simulink model "reacwheelfailure"  (R2014a)
settings: Solver=ode45  StartTime=0.0  StopTime=100.0  RelTol=1e-3
undefined symbols (not defined in the file): DiscIntNeverNeededParam, k, q1, q2, q3, q4
libraries: aerolibutil x2
settings Model: Creator=Gokull  LastModifiedBy=Gokull

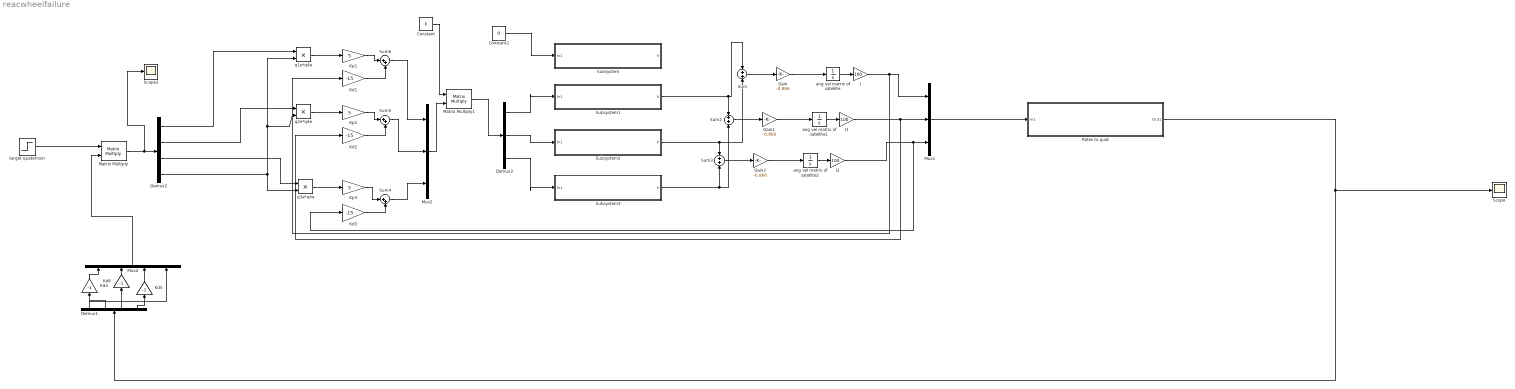
== system reacwheelfailure ==
  Constant : Constant  Value=k
  Constant1 : Constant  Value=0
  Demux1 : Demux
  Demux2 : Demux
  Demux3 : Demux  Outputs=3
  Gain : Gain  Gain=-0.866
  Gain1 : Gain  Gain=-0.866
  Gain2 : Gain  Gain=-0.866
  I : Gain  Gain=100
  I1 : Gain  Gain=100
  I2 : Gain  Gain=100
  Kd1 : Gain  Gain=-15
  Kd2 : Gain  Gain=-15
  Kd3 : Gain  Gain=-15
  Kd4 : Gain  Gain=-1
  Kd5 : Gain  Gain=-1
  Kd6 : Gain  Gain=-1
  Kp1 : Gain  Gain=5
  Kp2 : Gain  Gain=5
  Kp3 : Gain  Gain=5
  Matrix Multiply : Product  Multiplication=Matrix(*)
  Matrix Multiply1 : Product  Multiplication=Matrix(*)
  Mux1 : Mux  Inputs=3
  Mux2 : Mux  Inputs=3
  Mux4 : Mux
  Rates to quat : Subsystem
  Scope : Scope
      settings: TimeRange=600  YMin=-1  YMax=1  SaveName=ScopeData2
  Scope3 : Scope
      settings: SaveName=ScopeData3
  Subsystem : Subsystem
  Subsystem1 : Subsystem
  Subsystem2 : Subsystem
  Subsystem3 : Subsystem
  Sum : Sum  Inputs=+|+
  Sum2 : Sum  Inputs=+|+
  Sum3 : Sum  Inputs=+|+
  Sum4 : Sum  Inputs=|++
  Sum5 : Sum  Inputs=|++
  Sum6 : Sum  Inputs=|++
  ang vel matrix of satellite : Integrator
  ang vel matrix of satellite1 : Integrator
  ang vel matrix of satellite2 : Integrator
  q1e*q4e : Product
  q2e*q4e : Product
  q3e*q4e : Product
  target quaternion : Step  Before=[1,0,0,0;0,1,0,0;0,0,1,0;0,0,0,1]  After=[q4,q3,-q2,q1;-q3,q4,q1,q2;q2,-q1,q4,q3;-q1,-q2,-q3,q4]  SampleTime=0
  wires:
  Demux2/4 -> q1e*q4e/2, q2e*q4e/2, q3e*q4e/2
  q1e*q4e/1 -> Kp1/1
  q2e*q4e/1 -> Kp2/1
  q3e*q4e/1 -> Kp3/1
  Kp1/1 -> Sum6/1
  Kd1/1 -> Sum6/2
  Kp2/1 -> Sum5/1
  Kd2/1 -> Sum5/2
  Kp3/1 -> Sum4/1
  Kd3/1 -> Sum4/2
  Matrix Multiply/1 -> Scope3/1, Demux2/1
  Demux1/2 -> Kd4/1
  Demux1/3 -> Kd6/1
  Demux1/4 -> Kd5/1
  Demux1/1 -> Mux4/4
  target quaternion/1 -> Matrix Multiply/1
  Kd4/1 -> Mux4/1
  Kd6/1 -> Mux4/2
  Kd5/1 -> Mux4/3
  Mux4/1 -> Matrix Multiply/2
  Demux2/1 -> q1e*q4e/1
  Demux2/2 -> q2e*q4e/1
  Demux2/3 -> q3e*q4e/1
  Rates to quat/1(Out1) -> Demux1/1, Scope/1
  Subsystem3/1(h) -> Sum2/2, Sum3/2
  Subsystem1/1(h) -> Sum/1, Sum2/1
  Sum/1 -> Gain/1
  Gain/1 -> ang vel matrix of satellite/1
  ang vel matrix of satellite/1 -> I/1
  Mux1/1 -> Rates to quat/1(In1)
  Sum2/1 -> Gain1/1
  Gain1/1 -> ang vel matrix of satellite1/1
  ang vel matrix of satellite1/1 -> I1/1
  Sum3/1 -> Gain2/1
  Gain2/1 -> ang vel matrix of satellite2/1
  ang vel matrix of satellite2/1 -> I2/1
  Subsystem2/1(h) -> Sum/2, Sum3/1
  I1/1 -> Kd2/1, Mux1/2
  I/1 -> Kd1/1, Mux1/1
  I2/1 -> Kd3/1, Mux1/3
  Sum6/1 -> Mux2/1
  Sum5/1 -> Mux2/2
  Sum4/1 -> Mux2/3
  Constant/1 -> Matrix Multiply1/1
  Mux2/1 -> Matrix Multiply1/2
  Matrix Multiply1/1 -> Demux3/1
  Demux3/1 -> Subsystem1/1(In1)
  Demux3/2 -> Subsystem2/1(In1)
  Demux3/3 -> Subsystem3/1(In1)
  Constant1/1 -> Subsystem/1(In1)

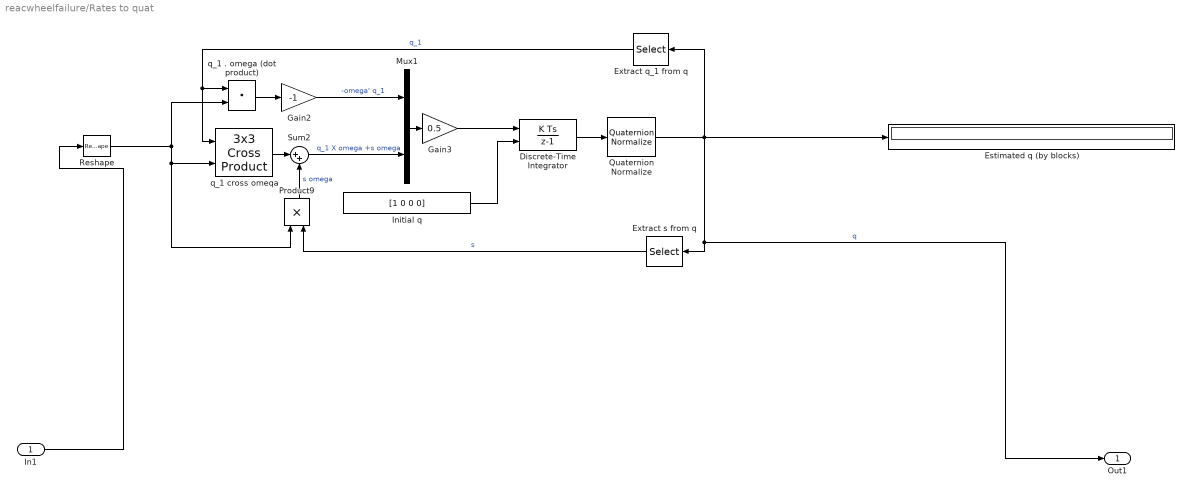
== system reacwheelfailure/Rates to quat ==
  In1 : Inport
  Discrete-Time Integrator : DiscreteIntegrator  InitialConditionSource=external  SampleTime=0.1  ICPrevOutput=DiscIntNeverNeededParam  ICPrevScaledInput=DiscIntNeverNeededParam
  Estimated q (by blocks) : Display
  Extract q_1 from q : Selector  InputPortWidth=4  Indices=[2:4]
  Extract s from q : Selector  InputPortWidth=4
  Gain2 : Gain  Gain=-1  SaturateOnIntegerOverflow=on  OutDataTypeStr=Inherit: Same as input  ParamDataTypeStr=Inherit: Same as input
  Gain3 : Gain  Gain=0.5  SaturateOnIntegerOverflow=on  OutDataTypeStr=Inherit: Same as input  ParamDataTypeStr=Inherit: Same as input
  "Initial q " : Constant  Value=[1 0 0 0]  VectorParams1D=off
  Mux1 : Mux  Inputs=2
  Product9 : Product  Inputs=**  SaturateOnIntegerOverflow=on  InputSameDT=on  OutDataTypeStr=Inherit: Same as first input
  Quaternion Normalize : aerolibutil/Quaternion Normalize
  Reshape : Reshape  OutputDimensionality=Row vector (2-D)
  Sum2 : Sum  Inputs=|++  SaturateOnIntegerOverflow=on
  q_1 . omega (dot product) : DotProduct  InputSameDT=on  OutDataTypeStr=Inherit: Inherit via internal rule
  q_1 cross omeqa : aerolibutil/3x3 Cross Product
  Out1 : Outport
  wires:
  Mux1/1 -> Gain3/1
  Quaternion Normalize/1 -> Out1/1, Extract s from q/1, Estimated q (by blocks)/1, Extract q_1 from q/1  "q"
  "Initial q "/1 -> Discrete-Time Integrator/2
  q_1 . omega (dot product)/1 -> Gain2/1
  Product9/1 -> Sum2/2  "s omega"
  Reshape/1 -> q_1 . omega (dot product)/2, q_1 cross omeqa/2, Product9/1
  q_1 cross omeqa/1 -> Sum2/1
  Sum2/1 -> Mux1/2  "q_1 X omega +s omega"
  Discrete-Time Integrator/1 -> Quaternion Normalize/1
  Gain2/1 -> Mux1/1  "-omega' q_1"
  Extract s from q/1 -> Product9/2  "s"
  Extract q_1 from q/1 -> q_1 cross omeqa/1, q_1 . omega (dot product)/1  "q_1"
  Gain3/1 -> Discrete-Time Integrator/1
  In1/1 -> Reshape/1

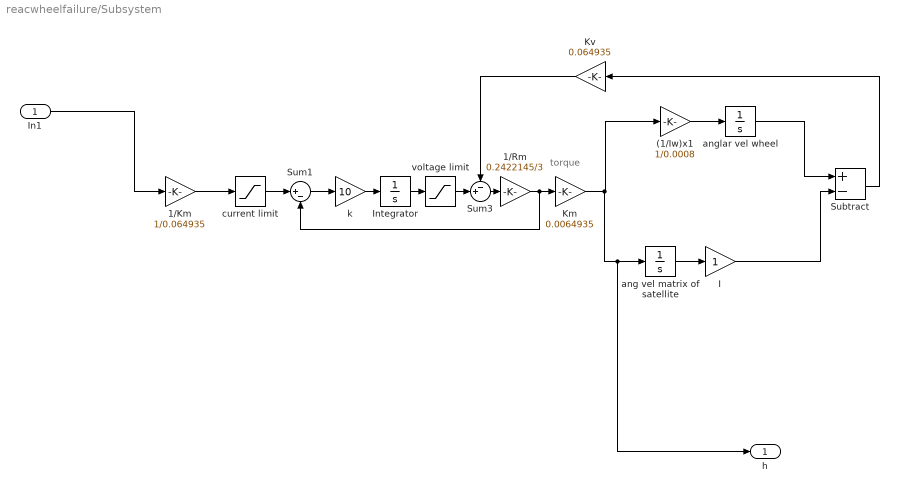
== system reacwheelfailure/Subsystem ==
  note: torque
  In1 : Inport
  (1/Iw)x1 : Gain  Gain=1/0.0008
  1/Km : Gain  Gain=1/0.064935
  1/Rm : Gain  Gain=0.2422145/3
  I : Gain
  Integrator : Integrator
  Km : Gain  Gain=0.0064935
  Kv : Gain  Gain=0.064935
  Subtract : Sum  Inputs=+-
  Sum1 : Sum  Inputs=|+-
  Sum3 : Sum  Inputs=-+|
  ang vel matrix of satellite : Integrator
  anglar vel wheel : Integrator
  current limit : Saturate  UpperLimit=0.8  LowerLimit=-0.8
  k : Gain  Gain=10
  voltage limit : Saturate  UpperLimit=35  LowerLimit=-35
  h : Outport
  wires:
  1/Km/1 -> current limit/1
  k/1 -> Integrator/1
  1/Rm/1 -> Sum1/2, Km/1
  current limit/1 -> Sum1/1
  Sum1/1 -> k/1
  Sum3/1 -> 1/Rm/1
  voltage limit/1 -> Sum3/2
  Integrator/1 -> voltage limit/1
  anglar vel wheel/1 -> Subtract/1
  Subtract/1 -> Kv/1
  I/1 -> Subtract/2
  (1/Iw)x1/1 -> anglar vel wheel/1
  In1/1 -> 1/Km/1
  Km/1 -> h/1, ang vel matrix of satellite/1, (1/Iw)x1/1
  Kv/1 -> Sum3/1
  ang vel matrix of satellite/1 -> I/1

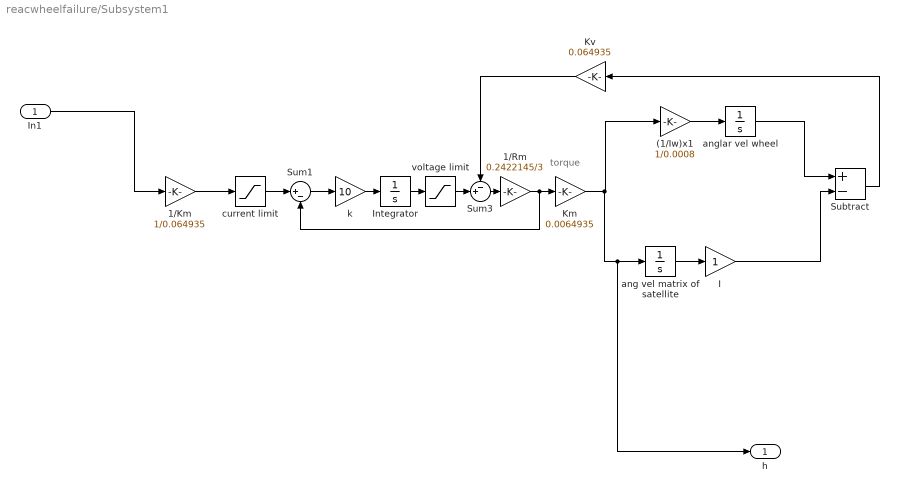
== system reacwheelfailure/Subsystem1 ==
  note: torque
  In1 : Inport
  (1/Iw)x1 : Gain  Gain=1/0.0008
  1/Km : Gain  Gain=1/0.064935
  1/Rm : Gain  Gain=0.2422145/3
  I : Gain
  Integrator : Integrator
  Km : Gain  Gain=0.0064935
  Kv : Gain  Gain=0.064935
  Subtract : Sum  Inputs=+-
  Sum1 : Sum  Inputs=|+-
  Sum3 : Sum  Inputs=-+|
  ang vel matrix of satellite : Integrator
  anglar vel wheel : Integrator
  current limit : Saturate  UpperLimit=0.8  LowerLimit=-0.8
  k : Gain  Gain=10
  voltage limit : Saturate  UpperLimit=35  LowerLimit=-35
  h : Outport
  wires:
  1/Km/1 -> current limit/1
  k/1 -> Integrator/1
  1/Rm/1 -> Sum1/2, Km/1
  current limit/1 -> Sum1/1
  Sum1/1 -> k/1
  Sum3/1 -> 1/Rm/1
  voltage limit/1 -> Sum3/2
  Integrator/1 -> voltage limit/1
  anglar vel wheel/1 -> Subtract/1
  Subtract/1 -> Kv/1
  I/1 -> Subtract/2
  (1/Iw)x1/1 -> anglar vel wheel/1
  In1/1 -> 1/Km/1
  Km/1 -> h/1, ang vel matrix of satellite/1, (1/Iw)x1/1
  Kv/1 -> Sum3/1
  ang vel matrix of satellite/1 -> I/1

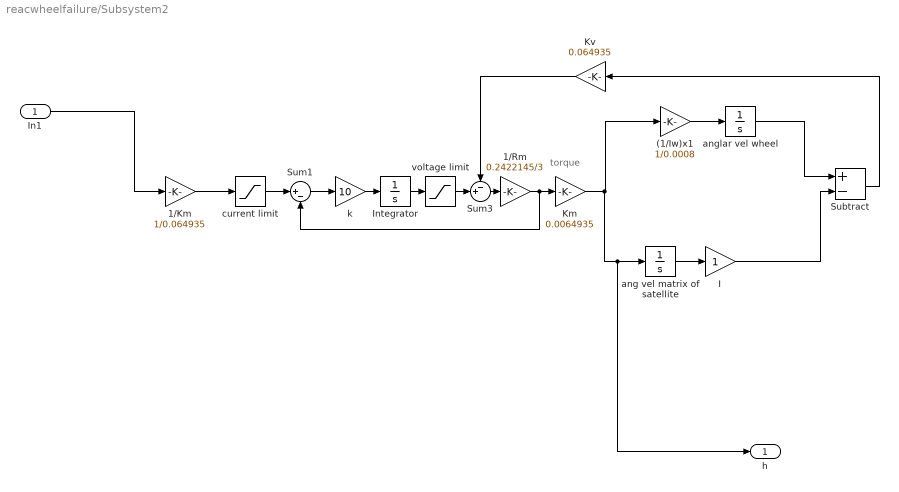
== system reacwheelfailure/Subsystem2 ==
  note: torque
  In1 : Inport
  (1/Iw)x1 : Gain  Gain=1/0.0008
  1/Km : Gain  Gain=1/0.064935
  1/Rm : Gain  Gain=0.2422145/3
  I : Gain
  Integrator : Integrator
  Km : Gain  Gain=0.0064935
  Kv : Gain  Gain=0.064935
  Subtract : Sum  Inputs=+-
  Sum1 : Sum  Inputs=|+-
  Sum3 : Sum  Inputs=-+|
  ang vel matrix of satellite : Integrator
  anglar vel wheel : Integrator
  current limit : Saturate  UpperLimit=0.8  LowerLimit=-0.8
  k : Gain  Gain=10
  voltage limit : Saturate  UpperLimit=35  LowerLimit=-35
  h : Outport
  wires:
  1/Km/1 -> current limit/1
  k/1 -> Integrator/1
  1/Rm/1 -> Sum1/2, Km/1
  current limit/1 -> Sum1/1
  Sum1/1 -> k/1
  Sum3/1 -> 1/Rm/1
  voltage limit/1 -> Sum3/2
  Integrator/1 -> voltage limit/1
  anglar vel wheel/1 -> Subtract/1
  Subtract/1 -> Kv/1
  I/1 -> Subtract/2
  (1/Iw)x1/1 -> anglar vel wheel/1
  In1/1 -> 1/Km/1
  Km/1 -> h/1, ang vel matrix of satellite/1, (1/Iw)x1/1
  Kv/1 -> Sum3/1
  ang vel matrix of satellite/1 -> I/1

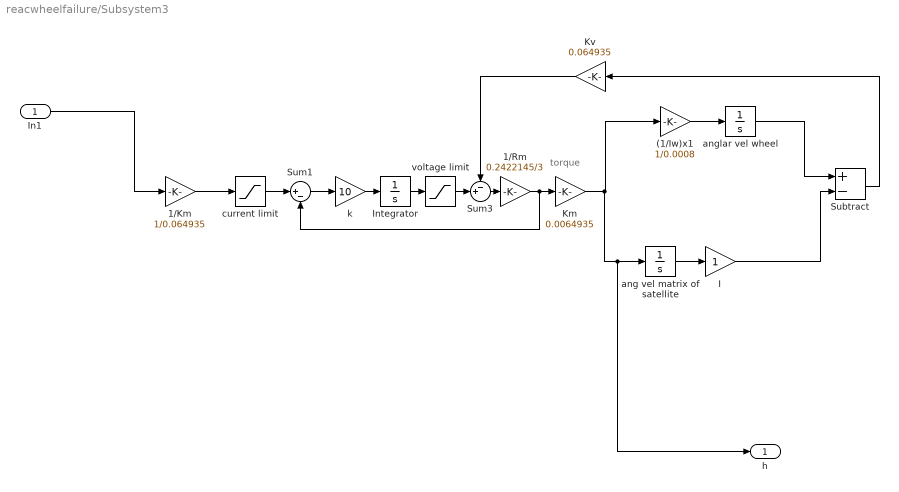
== system reacwheelfailure/Subsystem3 ==
  note: torque
  In1 : Inport
  (1/Iw)x1 : Gain  Gain=1/0.0008
  1/Km : Gain  Gain=1/0.064935
  1/Rm : Gain  Gain=0.2422145/3
  I : Gain
  Integrator : Integrator
  Km : Gain  Gain=0.0064935
  Kv : Gain  Gain=0.064935
  Subtract : Sum  Inputs=+-
  Sum1 : Sum  Inputs=|+-
  Sum3 : Sum  Inputs=-+|
  ang vel matrix of satellite : Integrator
  anglar vel wheel : Integrator
  current limit : Saturate  UpperLimit=0.8  LowerLimit=-0.8
  k : Gain  Gain=10
  voltage limit : Saturate  UpperLimit=35  LowerLimit=-35
  h : Outport
  wires:
  1/Km/1 -> current limit/1
  k/1 -> Integrator/1
  1/Rm/1 -> Sum1/2, Km/1
  current limit/1 -> Sum1/1
  Sum1/1 -> k/1
  Sum3/1 -> 1/Rm/1
  voltage limit/1 -> Sum3/2
  Integrator/1 -> voltage limit/1
  anglar vel wheel/1 -> Subtract/1
  Subtract/1 -> Kv/1
  I/1 -> Subtract/2
  (1/Iw)x1/1 -> anglar vel wheel/1
  In1/1 -> 1/Km/1
  Km/1 -> h/1, ang vel matrix of satellite/1, (1/Iw)x1/1
  Kv/1 -> Sum3/1
  ang vel matrix of satellite/1 -> I/1
